simulink model "model_simulink"  (R2017b)
settings: Solver=ode8  StartTime=0.0  StopTime=15  FixedStep=0.01  MaxStep=8.0  RelTol=1e-3
undefined symbols (not defined in the file): Serial_Port, Standard_Devices
libraries: simulink x3, sldrtlib x2
settings Model: Creator=Vjekoslav  LastModifiedBy=Vjekoslav
settings CodeAppCC: StateflowObjectComments=on

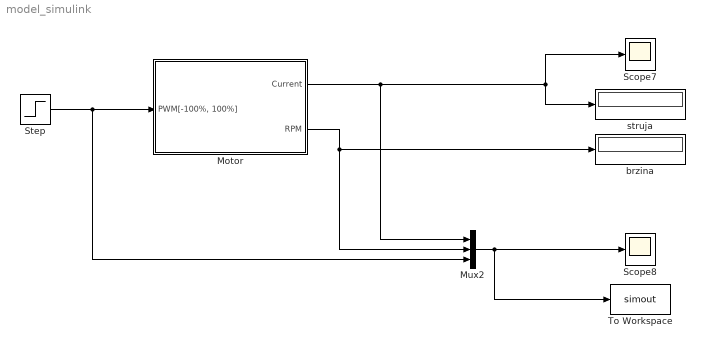
== system model_simulink ==
  Motor : Subsystem
  Mux2 : Mux  Inputs=3
  Scope7 : Scope
  Scope8 : Scope
  Step : Step  Time=10  Before=100  After=0  SampleTime=0
  To Workspace : ToWorkspace  VariableName=simout  SaveFormat=Timeseries  SampleTime=-1
  brzina : Display
  struja : Display
  wires:
  Mux2/1 -> To Workspace/1, Scope8/1
  Motor/1(Current) -> struja/1, Scope7/1, Mux2/1
  Motor/2(RPM) -> Mux2/2, brzina/1
  Step/1 -> Motor/1("PWM[-100%, 100%] "), Mux2/3
  ? -> ?

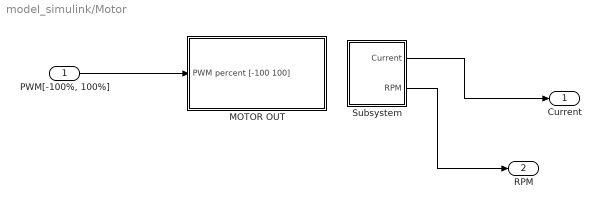
== system model_simulink/Motor ==
  "PWM[-100%, 100%] " : Inport
  MOTOR OUT : Subsystem
  Subsystem : Subsystem
  Current : Outport
  RPM : Outport  Port=2
  wires:
  "PWM[-100%, 100%] "/1 -> MOTOR OUT/1(PWM percent [-100 100])
  Subsystem/1(Current) -> Current/1
  Subsystem/2("RPM ") -> RPM/1

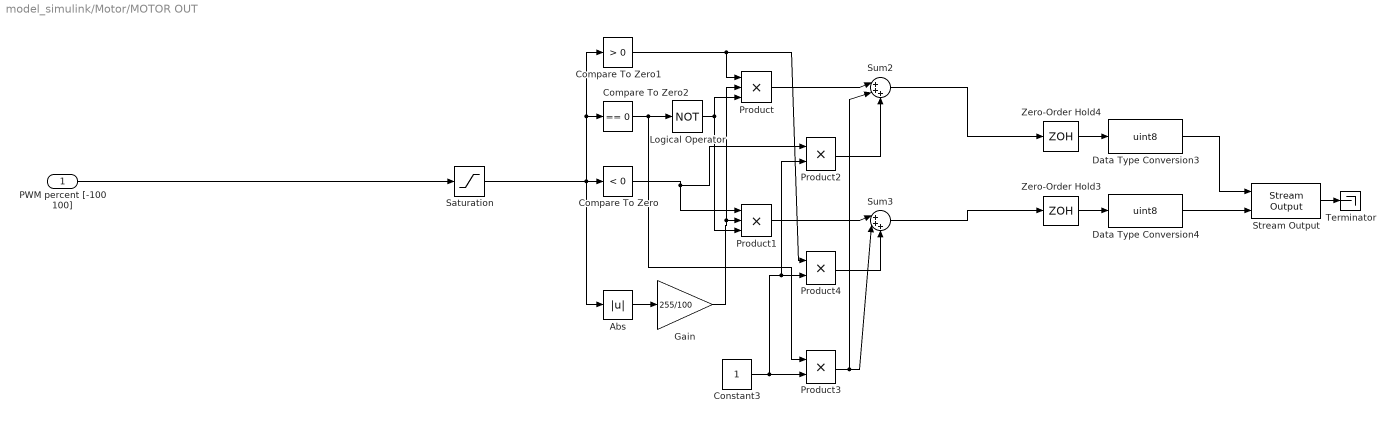
== system model_simulink/Motor/MOTOR OUT ==
  PWM percent [-100 100] : Inport
  Abs : Abs
  Compare To Zero : simulink/Logic and Bit Operations/Compare To Zero  relop=<  OutDataTypeStr=boolean
  Compare To Zero1 : simulink/Logic and Bit Operations/Compare To Zero  relop=>  OutDataTypeStr=boolean
  Compare To Zero2 : simulink/Logic and Bit Operations/Compare To Zero  relop===  OutDataTypeStr=boolean
  Constant3 : Constant
  Data Type Conversion3 : DataTypeConversion  OutMin=[0]  OutMax=[255]  OutDataTypeStr=uint8  RndMeth=Nearest
  Data Type Conversion4 : DataTypeConversion  OutMin=[0]  OutMax=[255]  OutDataTypeStr=uint8  RndMeth=Nearest
  Gain : Gain  Gain=255/100
  Logical Operator : Logic  Operator=NOT  AllPortsSameDT=off  OutDataTypeStr=boolean
  Product : Product  Inputs=3
  Product1 : Product  Inputs=3
  Product2 : Product
  Product3 : Product
  Product4 : Product
  Saturation : Saturate  UpperLimit=100  LowerLimit=-100
  Stream Output : sldrtlib/Stream Output  SampleTime=-1  MaxMissedTicks=inf  ShowMissedTicks=off  YieldWhenWaiting=off  DrvName=Standard_Devices/Serial_Port  DrvAddress=4  DrvOptions=[1000000 8 0 0 0 0 0 0]  PortSizes=[1 1]  FormatString='%c%c\n'  ShowReady=off  ShowError=on  InitialValue=[]  FinalValue=[]
      settings: AttributesFormatString=Standard Devices\nSerial Port [4h]  SourceProductName=Simulink Desktop Real-Time  SourceProductBaseCode=WT
  Sum2 : Sum  Inputs=|+++
  Sum3 : Sum  Inputs=|+++
  Terminator : Terminator
  Zero-Order Hold3 : ZeroOrderHold  SampleTime=-1
  Zero-Order Hold4 : ZeroOrderHold  SampleTime=-1
  wires:
  Product4/1 -> Sum3/3
  Product2/1 -> Sum2/3
  Logical Operator/1 -> Product/3, Product1/3
  Compare To Zero2/1 -> Product3/1, Logical Operator/1
  Product1/1 -> Sum3/1
  Sum3/1 -> Zero-Order Hold3/1
  Constant3/1 -> Product2/2, Product4/2, Product3/2
  Saturation/1 -> Abs/1, Compare To Zero1/1, Compare To Zero2/1, Compare To Zero/1
  Product3/1 -> Sum3/2, Sum2/2
  Compare To Zero1/1 -> Product4/1, Product/1
  Data Type Conversion3/1 -> Stream Output/1
  Zero-Order Hold3/1 -> Data Type Conversion4/1
  Gain/1 -> Product1/2, Product/2
  Abs/1 -> Gain/1
  Sum2/1 -> Zero-Order Hold4/1
  Zero-Order Hold4/1 -> Data Type Conversion3/1
  Compare To Zero/1 -> Product2/1, Product1/1
  Product/1 -> Sum2/1
  Data Type Conversion4/1 -> Stream Output/2
  Stream Output/1 -> Terminator/1
  PWM percent [-100 100]/1 -> Saturation/1

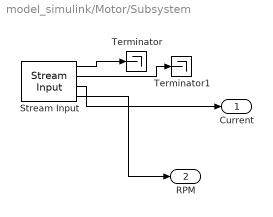
== system model_simulink/Motor/Subsystem ==
  Stream Input : sldrtlib/Stream Input  SampleTime=-1  MaxMissedTicks=inf  ShowMissedTicks=off  YieldWhenWaiting=off  DrvName=Standard_Devices/Serial_Port  DrvAddress=4  DrvOptions=[1000000 8 0 0 0 0 0 0]  DataTypes={'uint8' 'uint8' 'double' 'double'}  FormatString='%c%c\r%f\r%f'  Terminator='\n'  ShowReady=off  ShowError=off
      settings: AttributesFormatString=Standard Devices\nSerial Port [4h]  SourceProductName=Simulink Desktop Real-Time  SourceProductBaseCode=WT
  Terminator : Terminator
  Terminator1 : Terminator
  Current : Outport
  "RPM " : Outport  Port=2
  wires:
  Stream Input/3 -> Current/1
  Stream Input/4 -> "RPM "/1
  Stream Input/1 -> Terminator/1
  Stream Input/2 -> Terminator1/1
